simulink model "sm_car_test_Unreal_Engine_routing_by_version"  (R2023b)
settings: Solver=VariableStepAuto  StartTime=0.0  StopTime=10.0  RelTol=1e-3  AbsTol=1e-3
libraries: Vehicle_Visualization x1
Description:
  | Copyright 2020-2023 The MathWorks, Inc.
settings Model: Creator=smiller  LastModifiedBy=smiller
settings SolverCC: AutoScaleAbsTol=off  AlgebraicLoopSolver=TrustRegion
settings OptimizationCC: ReuseModelBlockBuffer=off
settings DebuggingCC: UnconnectedInputMsg=warning  UnconnectedOutputMsg=warning  UnconnectedLineMsg=warning  SymbolicDimsDataTypeCodeGenerationDiagnostic=none  ArithmeticOperatorsInVariantConditions=warning
settings ModelReferenceCC: EnableRefExpFcnMdlSchedulingChecks=on
settings SFSimCC: CustomCodeUndefinedFunction=UseInterfaceOnly
settings RTWCC: DLArmComputeVersion=19.05
settings SimscapeCC: SimscapeLogType=all  SimscapeLogSimulationStatistics=on  SimscapeLogDataHistory=10000

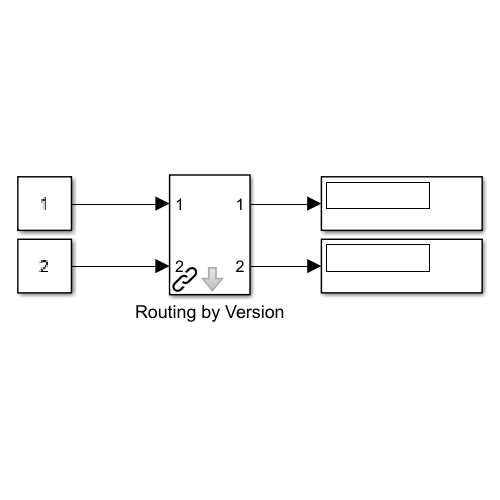
[thumbnail: Simulink's stored preview of the top-level diagram]
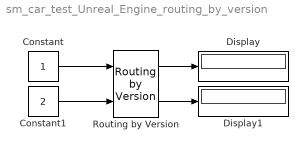
== system sm_car_test_Unreal_Engine_routing_by_version ==
  Constant : Constant
  Constant1 : Constant  Value=2
  Display : Display
  Display1 : Display
  Routing by Version : Vehicle_Visualization/Routing by Version  post_19a=-1
  wires:
  Routing by Version/1 -> Display/1
  Routing by Version/2 -> Display1/1
  Constant/1 -> Routing by Version/1
  Constant1/1 -> Routing by Version/2
